simulink library "SignalPreprocessingLib"  (R2020b)
settings: Solver=VariableStepAuto  StartTime=0.0  StopTime=10.0  RelTol=1e-3
undefined symbols (not defined in the file or in its folder): fdesignblkfcn, fs, gcbh, param_ecg_gain_mv
(part 7 of 7)

== system SignalPreprocessingLib/SCGxyz Gain + Filtfilter/Enabled SCG Preprocessing Subsystem/Filtfiltering/Bandpass Filter 2 ==
  In : Inport
  Generated Filter Block : DiscreteFir  Tag=BlockMethodSubSystem  Coefficients=[-0.00978480817658220967 0.00796999512757378195 0.00147001916949950507 -0.00206976963634554088 -0.00243890991203639124 -0.000924134149517863001 0.000721734906664772908 0.00129711475091687537 0.000656253913654551951 -0.000505332991406271686 -0.0012801272291147899 -0.00118584056106384888 -0.000396379626042962676 0.000462570629011344568 0.00079523934067100995 0.000413152706797699921 -0.000373518377931415205 -0.00101662167067520059 -0.00109601261216027662 -0.000593906547902721513 0.00013435029468211794 0.000600271945192065227 0.000514574052205835205 -5.24294882560059138e-05 -0.000721006732064664153 -0.00106936812684002851 -0.000885784329198623685 -0.000306368867510058802 0.000299921121108211923 0.00055090300805175213 0.000305129539032457354 -0.000280348626867030323 -0.000834835852168314672 -0.00102988416243328038 -0.000749730060181843442 -0.00018384442768847384 0.000330781953284531652 0.000474456713548894286 0.00018715851511990093 -0.00037570651628371528 -0.000841441599320687434 -0.000980583400496216851 -0.000677521760008558955 -0.000143136714861572342 0.000296905261906841298 0.000427455994318532166 0.00013698321512635404 -0.000377779512805234978 -0.000807928899011485448 -0.000914634913299251437 -0.000653887485439495482 -0.000162386642357020724 0.000270410746944910174 0.000394818020750343026 0.000144292032000806675 -0.000318126126834723073 -0.000730717848545356027 -0.000862982022422141819 -0.0006461832253515002 -0.000197068691395214035 0.000227657437070046339 0.000390339376955589645 0.000202019386221156732 -0.000218262841065524645 -0.000630398467646775583 -0.000802033681634044845 -0.000643386601296857597 -0.000239583998883231527 0.000186056910795609839 0.000403403846243817683 0.000291609858585275487 -8.00732001476186567e-05 -0.000501540638877951057 -0.000730203151559393848 -0.000640276523076700071 -0.00027737553443828801 0.000156493764593411161 0.00043156139543532344 0.000397367103231359312 8.29189622619686553e-05 -0.000340599175797182173 -0.000631305624859686211 -0.000622947681400518255 -0.000317342453511192167 0.000133455335091144057 0.000471287365522237995 0.000526528964862326278 0.000266844016988408261 -0.000160112953992838734 -0.000507941523151940531 -0.000580953412745898053 -0.000334693556591401226 0.000109719501491407223 0.000513360648349098832 0.000657877410860213761 0.000469632889523299087 5.66691264257968493e-05 -0.00035174600552400606 -0.000520266671698473124 -0.000342073082939085209 9.47970697972318443e-05 0.000556210436752066603 0.000795382016377131282 0.000685450046798985143 0.000289752333424098715 -0.000168394924182923401 -0.000424984820321057985 -0.000326854493347916676 8.34347145894279147e-05 0.000590237414229303711 0.000924037851917966133 0.000905501272637524823 0.000546953829290044167 5.01002670594704154e-05 -0.000300380671439964494 -0.00029725255069634499 7.24448185066152141e-05 0.000616892125763008367 0.00104469796439719061 0.0011254010687403752 0.000815941579190399566 0.000293722454277149864 -0.000147131313195571635 -0.000243553418517324018 6.68821353140179397e-05 0.000631331563725699208 0.00114457781901217874 0.00133020230521578835 0.00109202570585933685 0.000561661563459188678 4.12191178191941113e-05 -0.000168825603708367067 6.18472916977904128e-05 0.000623699245113693902 0.00121794150913768183 0.0015200947806226976 0.00136753539574389362 0.000847811546795603659 0.000253069734210485946 -7.61054743145556534e-05 5.94169316983781721e-05 0.000599709927775937484 0.00125856843564240545 0.00167936422330872853 0.00163112458376294235 0.00114116904428636801 0.000486071978403662479 3.87954501406567137e-05 5.99888187065994788e-05 0.000552926215869422081 0.00125934973898075798 0.00179616995776612381 0.00186851973153335919 0.00143595292525184009 0.000740124310155826576 0.000171789154674743978 5.84203269058169574e-05 0.000478305096295934275 0.00121446318353966051 0.00186532763417856444 0.00207320507044359784 0.00171914297636467346 0.0010007500900107956 0.000316849149570202051 5.78099051728010543e-05 ...(+13942 chars)]  InputProcessing=Columns as channels (frame based)
  Out : Outport  VectorParamsAs1DForOutWhenUnconnected=off
  wires:
  In/1 -> Generated Filter Block/1
  Generated Filter Block/1 -> Out/1

== system SignalPreprocessingLib/SCGxyz Gain + Filtfilter/Enabled SCG Preprocessing Subsystem/To Workspace: Gain + Filtfiltered SCGxyz/To Workspace Enabled Subsystem ==
  note: The subsystem is only enabled when it receives a (non-zero) signal
  In1 : Inport
  Enable : EnablePort
  To Workspace Gain + Filtfiltered SCGxyz : ToWorkspace  VariableName=out_gain_filfiltered_scgxyz  SaveFormat=Structure  SampleTime=-1
  wires:
  In1/1 -> To Workspace Gain + Filtfiltered SCGxyz/1

== matlab function SignalPreprocessingLib/Generic Gain + Filtfilter/Enabled Sig Preprocessing Subsystem/Enabled Subsystem/Plotting ==
  data: preprocessed_sig input size=[param_tot_samples 1]; raw_sig input size=[param_tot_samples 1]; fs input size=[1]
function slk_wrapped_plotting_preprocessed_sig(preprocessed_sig, raw_sig, fs)
    
coder.extrinsic('plotting_preprocessed_sig');

if preprocessed_sig % Only go into the function if a valid (non-zero) signal is passed to it.
    plotting_preprocessed_sig(preprocessed_sig, raw_sig, fs)
end

end

== matlab function SignalPreprocessingLib/FiltFilter/Enabled Filtfiltering Subsystem/Plotting/Plotting ==
  data: filtfiltered_sig input size=[param_tot_samples 1]; raw_sig input size=[param_tot_samples 1]; fs input size=[1]
function slk_wrapped_plotting_preprocessed_sig(filtfiltered_sig, raw_sig, fs)
    
coder.extrinsic('plotting_preprocessed_sig');

if filtfiltered_sig % Only go into the function if a valid (i.e. non-zero) signal is passed to it.
    plotting_preprocessed_sig(filtfiltered_sig, raw_sig, fs)
end

end

== matlab function SignalPreprocessingLib/ECG Gain + Filtfilter/Enabled ECG Preprocessing Subsystem/Subsystem/Plotting ==
  data: preprocessed_ecg input size=[param_tot_samples 1]; raw_ecg input size=[param_tot_samples 1]; fs input size=[1]
function slk_wrapped_plotting_preprocessed_ecg(preprocessed_ecg, raw_ecg, fs)
    
coder.extrinsic('plotting_preprocessed_ecg');

if preprocessed_ecg % Only go into the function if a valid ecg R peak sequence is passed to it.
    plotting_preprocessed_ecg(preprocessed_ecg, raw_ecg, fs)
end

end

== matlab function SignalPreprocessingLib/SCGxyz Gain + Filtfilter/Enabled SCG Preprocessing Subsystem/Plotting/Plotting ==
  data: gain_filtfiltered_scg_xyz input size=[param_tot_samples 3]; raw_scg_xyz input size=[param_tot_samples 3]; fs input size=[1]
function slk_wrapped_plotting_preprocessed_scg_xyz(gain_filtfiltered_scg_xyz, raw_scg_xyz, fs)
    
coder.extrinsic('plotting_preprocessed_scg_xyz');

if gain_filtfiltered_scg_xyz(:,1) % Only go into the function if a valid ecg R peak sequence is passed to it.
    plotting_preprocessed_scg_xyz(gain_filtfiltered_scg_xyz, raw_scg_xyz, fs);
end

end
